simulink model "Problem_No5"  (R2020a)
settings: Solver=VariableStepAuto  StartTime=0.0  StopTime=10  MaxStep=0.01  RelTol=1e-3
model workspace (MAT data in the model file):
  C = Simulink.Parameter
  C.Value = 1e-05
  C.DataType = 'auto'
  C.Dimensions = [1 1]
  R = Simulink.Parameter
  R.Value = 10
  R.DataType = 'auto'
  R.Dimensions = [1 1]
settings Model: Creator='Z'ome  LastModifiedBy='Z'ome

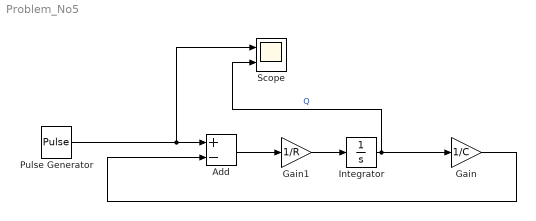
== system Problem_No5 ==
  Add : Sum  Inputs=+-
  Gain : Gain  Gain=1/C
  Gain1 : Gain  Gain=1/R
  Integrator : Integrator  InitialCondition=5
  Pulse Generator : DiscretePulseGenerator  PulseType=Time based  Amplitude=5  Period=5  PulseWidth=50
  Scope : Scope  NumInputPorts=2
  wires:
  Integrator/1 -> Scope/2, Gain/1  "Q"
  Gain/1 -> Add/2
  Gain1/1 -> Integrator/1
  Add/1 -> Gain1/1
  Pulse Generator/1 -> Scope/1, Add/1
